simulink model "can_simple_block_bu11143"  (R2016b)
settings: Solver=FixedStepDiscrete  StartTime=0.0  StopTime=1000  FixedStep=0.2  RelTol=1e-3  EnableMultiTasking=on
undefined symbols (not defined in the file or in its folder): A, A10, A14, B, B11, B12, B13, B8, C, CS0, CS1, D, D11, D4, F3, F4, G, G3, G4, H3, H4, K17, K4, L3, N16, PA11, PA12, PD0, PE14, PE15, R10, R14, R17, SCK, SIN, SOUT, T14
libraries: rappid_564xl_ec_toolbox x59
(part 1 of 6)
settings Model: Creator=RMuradov  LastModifiedBy=eugkim01
settings SolverCC: AutoInsertRateTranBlk=on
settings DataIOCC: ExternalInput=off  InitialState=off  LimitDataPoints=on  SaveFormat=Array  SignalLoggingSaveFormat=ModelDataLogs  SaveOutput=off  SignalLogging=off  SaveTime=off
settings OptimizationCC: DefaultParameterBehavior=Inlined  UseDivisionForNetSlopeComputation=on  UseFloatMulNetSlope=on  UseSpecifiedMinMax=on  InlineInvariantSignals=on  PassReuseOutputArgsAs=Individual arguments  ExpressionDepthLimit=2147483647  ZeroExternalMemoryAtStartup=off  ZeroInternalMemoryAtStartup=off  NoFixptDivByZeroProtection=on  EfficientFloat2IntCast=on  LifeSpan=1
settings DebuggingCC: UnderspecifiedInitializationDetection=Classic  MergeDetectMultiDrivingBlocksExec=none  SolverPrmCheckMsg=warning  InheritedTsInSrcMsg=none  SingleTaskRateTransMsg=error  ParameterTunabilityLossMsg=error  FcnCallInpInsideContextMsg=warning  UnconnectedInputMsg=error  UnconnectedOutputMsg=error  UnconnectedLineMsg=error  UnknownTsInhSupMsg=error  StateNameClashWarn=warning  SFUnexpectedBacktrackingDiag=warning  SFNoUnconditionalDefaultTransitionDiag=warning  SFExecutionAtInitializationDiag=none
settings HardwareCC: ProdBitPerPointer=32  ProdBitPerSizeT=32  ProdBitPerPtrDiffT=32  ProdLargestAtomicInteger=Long  ProdLargestAtomicFloat=Double  ProdEndianess=BigEndian  ProdWordSize=32  ProdHWDeviceType=Freescale->32-bit PowerPC
settings ModelReferenceCC: PropagateSignalLabelsOutOfModel=off
settings RTWCC: SystemTargetFile=rappid564xl.tlc  MakeCommand=rappid_564xl_make_rtw  TemplateMakefile=rappid_564xl_default_tmf  PostCodeGenCommand=rappid_analyzegencode(buildInfo)  Description=RAppID Toolbox MPC564xL Code Generation Target (rappid)  GenerateReport=on  TLCAssert=on  BuildConfiguration=Faster Runs  IncludeHyperlinkInReport=on  LaunchReport=on  GenerateTraceInfo=on  GenerateTraceReport=on  GenerateTraceReportSl=on  GenerateTraceReportSf=on  GenerateTraceReportEml=on  GenerateCodeMetricsReport=on
settings CodeAppCC: ForceParamTrailComments=on  IgnoreCustomStorageClasses=off  OperatorAnnotations=on  SimulinkDataObjDesc=on  SFDataObjDesc=on  MATLABFcnDesc=on  CustomSymbolStrGlobalVar=rt$N$M  CustomSymbolStrType=$N$M  CustomSymbolStrFcn=$N$M$F  CustomSymbolStrMacro=$N$M  InsertBlockDesc=on  MATLABSourceComments=on  InternalIdentifier=Classic
settings STFCustomTargetCC: CombineOutputUpdateFcns=on  CombineSignalStateStructs=on  SuppressErrorStatus=on  ERTCustomFileBanners=on  SupportAbsoluteTime=off  SupportNonFinite=off  SupportComplex=off  SupportContinuousTime=off  RemoveResetFunc=on  SupportVariableSizeSignals=on  MATLABClassNameForMDSCustomization=Simulink.SoftwareTarget.ERTCustomization  GRTInterface=off  SystemTargetFile=rappid564xl.tlc
settings ERTTargetCC: ParMdlRefBuildCompliant=off  CompOptLevelCompliant=off  ConcurrentExecutionCompliant=off  CombineSignalStateStructs=on  SuppressErrorStatus=on  ERTFirstTimeCompliant=off  SupportAbsoluteTime=off  SupportNonFinite=off  SupportComplex=off  SupportNonInlinedSFcns=on  SupportVariableSizeSignals=on  ModelStepFunctionPrototypeControlCompliant=off  CPPClassGenCompliant=off  UseToolchainInfoCompliant=off  InlinedParameterPlacement=NonHierarchical  ERTCustomFileTemplate=example_file_process.tlc
settings ConfigComp: CovMetricSettings=dw  CovHtmlReporting=on  CovSaveCumulativeToWorkspaceVar=on  CovSaveSingleToWorkspaceVar=on  CovExternalEMLEnable=off

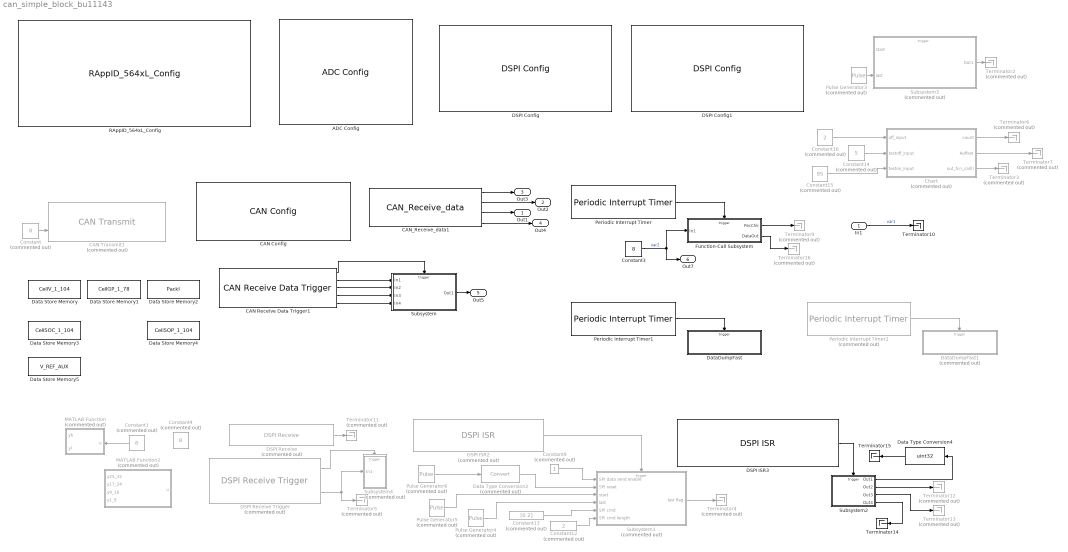
== system can_simple_block_bu11143 ==
  In1 : Inport
  ADC Config : rappid_564xl_ec_toolbox/MPC564xL/Motor Control Blocks/ADC Config  adc_unit=0  adc_ctu=off  adc_owr=on  adc_wls=Left  adc_clk=on  adc_ack=on  adc_ctr0_inp=off  adc_ctr0_shft=10 - Avin = 0  adc_ctr0_cmp=01  adc_ctr0_samp=3  adc_ctr1_inp=off  adc_ctr1_cmp=01  adc_ctr1_samp=1  adc_ctr1_tsens=PTAT  adc_pscr_preval=V0  adc_pscr_preconv=off
  CAN Config : rappid_564xl_ec_toolbox/MPC564xL/Communication Blocks/CAN Config  Priority=1  can_unit=A  can_unit_v2=0  can_idam=A - One full ID (standard or extended) per filter element.  can_srx_dis=1 - Self reception disabled  can_presdiv=4  can_rjw=3  can_pseg1=3  can_pseg2=3  can_clk_src=0 - The CAN engine clock source is the oscillator clock  can_lpb=0 - Loop Back disabled  can_smp=1 - Three samples are used to determine the value of the received bit  can_boff_rec=0 - Automatic recovering from Bus Off state enabled  can_tsyn=0 - Timer Sync feature disabled  can_lbuf=0 - Buffer with highest priority is transmitted first  can_lom=0 - Listen Only Mode is deactivated  can_propseg=6
  CAN Receive Data Trigger1 : rappid_564xl_ec_toolbox/MPC564xL/Communication Blocks/CAN Receive Data Trigger  can_unit=A  can_unit_v2=0  can_buffer=5  can_id=1021  can_isr_prio=14
  CAN Transmit1 : rappid_564xl_ec_toolbox/MPC564xL/Communication Blocks/CAN Transmit  Commented=on  can_unit=A  can_unit_v2=0  can_buffer=14  can_id=522
  CAN_Receive_data1 : rappid_564xl_ec_toolbox/MPC564xL/Communication Blocks/CAN_Receive_data  can_unit=A  can_unit_v2=0  can_buffer=7  can_id=1010
  Chart : Stateflow chart  Commented=on  TreatAsAtomicUnit=on
  Constant : Constant  Commented=on  Value=8  OutDataTypeStr=uint8
  Constant1 : Constant  Commented=on  Value=8  OutDataTypeStr=uint16
  Constant12 : Constant  Commented=on  Value=2  OutDataTypeStr=uint8
  Constant13 : Constant  Commented=on  Value=[0 2]  OutDataTypeStr=uint8
  Constant14 : Constant  Commented=on  Value=5
  Constant15 : Constant  Commented=on  Value=95
  Constant16 : Constant  Commented=on  Value=2
  Constant3 : Constant  Value=8  OutDataTypeStr=uint16
  Constant4 : Constant  Commented=on  Value=8  OutDataTypeStr=uint16
  Constant9 : Constant  Commented=on  OutDataTypeStr=boolean
  DSPI Config : rappid_564xl_ec_toolbox/MPC564xL/Communication Blocks/DSPI Config  Priority=1  dspi_Num=1  dspi_Mode=Master  dspi_MTFE=off  dspi_CONT_SCKE=off  dspi_PCSSE=off  dspi_ROOE=off  dspi_DIS_TXF=Disable  dspi_DIS_RXF_v2=Disable  dspi_SMPL_PT=DSPI samples SIN at driving SCK edge  dspi_FMSZ=8  dspi_CPOL=High  dspi_CPHA=Data is changed on the leading edge of SCK and captured on the following edge  dspi_LSBFE=MSB first  dspi_DBR=off  dspi_PCSSCK=7  dspi_PASC=1  dspi_PDT=5  dspi_PBR=3  dspi_CSSCK=256  dspi_ASC=256  dspi_DT=8  dspi_BR=64  dspi_PCSIS0=High  dspi_PCSIS1=High  dspi_PCSIS2=High  dspi_PCSIS3=High  dspi_PCSIS4=High  dspi_PCSIS5=High  dspi_PCSIS6=High  dspi_PCSIS7=High  dspi_DIS_RXF=Oops
  DSPI Config1 : rappid_564xl_ec_toolbox/MPC564xL/Communication Blocks/DSPI Config  Priority=1  dspi_Num=0  dspi_Mode=Master  dspi_MTFE=off  dspi_CONT_SCKE=off  dspi_PCSSE=off  dspi_ROOE=off  dspi_DIS_TXF=Disable  dspi_DIS_RXF_v2=Disable  dspi_SMPL_PT=DSPI samples SIN at driving SCK edge  dspi_FMSZ=8  dspi_CPOL=High  dspi_CPHA=Data is changed on the leading edge of SCK and captured on the following edge  dspi_LSBFE=MSB first  dspi_DBR=off  dspi_PCSSCK=7  dspi_PASC=1  dspi_PDT=5  dspi_PBR=3  dspi_CSSCK=256  dspi_ASC=256  dspi_DT=8  dspi_BR=64  dspi_PCSIS0=High  dspi_PCSIS1=High  dspi_PCSIS2=High  dspi_PCSIS3=High  dspi_PCSIS4=High  dspi_PCSIS5=High  dspi_PCSIS6=High  dspi_PCSIS7=High  dspi_DIS_RXF=Oops
  DSPI ISR2 : rappid_564xl_ec_toolbox/MPC564xL/Communication Blocks/DSPI ISR  Commented=on  dspi_Num=1  dspi_isr_name=TCF - Transfer Complete  dspi_isrPrio=13  dspi_isr_tfuf=off  dspi_isr_rfof=on
  DSPI ISR3 : rappid_564xl_ec_toolbox/MPC564xL/Communication Blocks/DSPI ISR  dspi_Num=1  dspi_isr_name=EOQF - End of Queue  dspi_isrPrio=11  dspi_isr_tfuf=off  dspi_isr_rfof=on
  DSPI Receive : rappid_564xl_ec_toolbox/MPC564xL/Communication Blocks/DSPI Receive  Commented=on  dspi_Num=1
  DSPI Receive Trigger : rappid_564xl_ec_toolbox/MPC564xL/Communication Blocks/DSPI Receive Trigger  Commented=on  dspi_Num=1  dspi_ISRPri=13
  Data Store Memory : DataStoreMemory  DataStoreName=CellV_1_104  ReadBeforeWriteMsg=warning  WriteAfterWriteMsg=warning  WriteAfterReadMsg=warning  ShowAdditionalParam=off  OutDataTypeStr=uint16  Dimensions=104
  Data Store Memory1 : DataStoreMemory  DataStoreName=CellGP_1_78  ReadBeforeWriteMsg=warning  WriteAfterWriteMsg=warning  WriteAfterReadMsg=warning  ShowAdditionalParam=off  OutDataTypeStr=uint16  Dimensions=78
  Data Store Memory2 : DataStoreMemory  DataStoreName=PackI  ReadBeforeWriteMsg=warning  WriteAfterWriteMsg=warning  WriteAfterReadMsg=warning  ShowAdditionalParam=off  OutDataTypeStr=int32  Dimensions=1
  Data Store Memory3 : DataStoreMemory  DataStoreName=CellSOC_1_104  ReadBeforeWriteMsg=warning  WriteAfterWriteMsg=warning  WriteAfterReadMsg=warning  ShowAdditionalParam=off  OutDataTypeStr=uint16  Dimensions=104
  Data Store Memory4 : DataStoreMemory  DataStoreName=CellSOP_1_104  ReadBeforeWriteMsg=warning  WriteAfterWriteMsg=warning  WriteAfterReadMsg=warning  ShowAdditionalParam=off  OutDataTypeStr=int16  Dimensions=104
  Data Store Memory5 : DataStoreMemory  DataStoreName=V_REF_AUX  ReadBeforeWriteMsg=warning  WriteAfterWriteMsg=warning  WriteAfterReadMsg=warning  InitialValue=3  ShowAdditionalParam=off  OutDataTypeStr=uint16  Dimensions=1
  Data Type Conversion2 : DataTypeConversion  Priority=1  Commented=on
  Data Type Conversion4 : DataTypeConversion  Priority=1  OutDataTypeStr=uint32
  DataDumpFast : Subsystem  TreatAsAtomicUnit=on
      settings: RTWSystemCode=Nonreusable function
  DataDumpFast1 : Subsystem  Commented=on  TreatAsAtomicUnit=on
      settings: RTWSystemCode=Nonreusable function
  Function-Call Subsystem : Subsystem  TreatAsAtomicUnit=on
      settings: RTWSystemCode=Nonreusable function
  MATLAB Function : MATLAB Function  Commented=on  TreatAsAtomicUnit=on
  MATLAB Function2 : MATLAB Function  Commented=on  TreatAsAtomicUnit=on
  Periodic Interrupt Timer : rappid_564xl_ec_toolbox/MPC564xL/General Purpose Blocks/Periodic Interrupt Timer  pit_chan=1  pit_timeout=50  int_priority=12  pit_timeout_val=5999999
  Periodic Interrupt Timer1 : rappid_564xl_ec_toolbox/MPC564xL/General Purpose Blocks/Periodic Interrupt Timer  pit_chan=2  pit_timeout=10  int_priority=13  pit_timeout_val=1199999
  Periodic Interrupt Timer2 : rappid_564xl_ec_toolbox/MPC564xL/General Purpose Blocks/Periodic Interrupt Timer  Commented=on  pit_chan=2  pit_timeout=100  int_priority=13  pit_timeout_val=11999999
  Pulse Generator3 : DiscretePulseGenerator  Commented=on  Period=100  PhaseDelay=5
  Pulse Generator4 : DiscretePulseGenerator  Commented=on  Period=100  PhaseDelay=5
  Pulse Generator5 : DiscretePulseGenerator  Commented=on  Period=100
  Pulse Generator6 : DiscretePulseGenerator  Commented=on  Period=10000000  PhaseDelay=1
  RAppID_564xL_Config : rappid_564xl_ec_toolbox/MPC564xL/RAppID_564xL_Config  SystemClock=120  XTAL=40  MC_clock_60=12  MC_clock_80=16  MC_clock_120=10  SWG_clock_60=20  SWG_clock_80=13.334  SWG_clock_120=20  Compiler=CodeWarrior  MemTarget=FLASH  Part=MPC5643L  Package=144 LQFP  global_int_priority=11  base_tick_priority=12  sys_task_supress=off  exception_handlers=off  stored_mdl_name=can_simple_block_bu11142  freemaster_interface=Oops  freemaster_rx_pin="LINFlex_0 Rx Pin 116 : \"PB[3]\""  freemaster_tx_pin="LINFlex_0 Tx Pin 114 : \"PB[2]\""  freemaster_interface_1=None  freemaster_enable=off  freemaster_rate=57600  freemaster_tx0_pin=18 : B[2] : 114 : A14  freemaster_rx0_pin=19 : B[3] : 116 : B13  freemaster_tx1_pin=57 : D[9] : 26 : L3  freemaster_rx1_pin=29 : B[13] : 60 : R10  freemaster_can_channel=1CH  freemater_can_speed=500K  freemaster_can_msgig=0x7AA  ccp_interface=None  ccp_enable=off  ccp_can_channel=CH1 (MB 0 - 1)  ccp_can_speed=500K  ccp_can_cro_id=256  ccp_can_dto_id=257  ccp_dev_id=RappID  ccp_dev_addr=0  ccp_odt=3  ccp_daq=3  pil_enable=off  pil_bam=off  comport=6  pil_rate=57600  bam_password_def=on  bam_password=0xFEEDFACECAFEBEEF  bam_sa_cs=on  bam_start_address=0x40005000  bam_code_size=0xa000  cons_dspi=on  cons_can=on  cons_adc=on  cons_pwm=on  cons_ctu=on  cons_swg=on  cons_eTimer=on  cons_fm=on
  Subsystem : Subsystem
      settings: RTWSystemCode=Nonreusable function
  Subsystem1 : Subsystem  Commented=on
      settings: RTWSystemCode=Nonreusable function
  Subsystem2 : Subsystem
      settings: RTWSystemCode=Nonreusable function
  Subsystem3 : Subsystem  Commented=on
  Subsystem4 : Subsystem  Commented=on
      settings: RTWSystemCode=Nonreusable function
  Terminator10 : Terminator
  Terminator{2..7,9,11..13,16} (11 alike) : Terminator  Commented=on
  Terminator14 : Terminator
  Terminator15 : Terminator
  Out1 : Outport
  Out2 : Outport  Port=2
  Out3 : Outport  Port=3
  Out4 : Outport  Port=4
  Out5 : Outport  Port=5
  Out7 : Outport  Port=6
  wires:
  CAN_Receive_data1/4 -> Out4/1
  CAN_Receive_data1/3 -> Out1/1
  CAN_Receive_data1/2 -> Out2/1
  CAN_Receive_data1/1 -> Out3/1
  Constant/1 -> CAN Transmit1/2
  CAN Receive Data Trigger1/3 -> Subsystem/2(In2)
  CAN Receive Data Trigger1/4 -> Subsystem/3(In3)
  CAN Receive Data Trigger1/5 -> Subsystem/4(In4)
  CAN Receive Data Trigger1/2 -> Subsystem/1(In1)
  CAN Receive Data Trigger1/1 -> Subsystem/Trigger
  Subsystem/1(Out1) -> Out5/1
  DSPI ISR2/1 -> Subsystem1/Trigger
  DSPI ISR3/1 -> Subsystem2/Trigger
  Constant9/1 -> Subsystem1/1(SPI data send enable)
  Subsystem1/1(last flag) -> Terminator4/1
  Pulse Generator3/1 -> Subsystem3/2(last)
  Subsystem3/1(Out1) -> Terminator2/1
  Pulse Generator4/1 -> Subsystem1/4(last)
  Constant12/1 -> Subsystem1/6(SPI cmd length)
  Constant13/1 -> Subsystem1/5(SPI cmd)
  Chart/1(count) -> Terminator6/1
  Chart/2(" Aoffset") -> Terminator7/1
  Constant16/1 -> Chart/1(off_input)
  Constant14/1 -> Chart/2(testoff_input)
  Constant15/1 -> Chart/3(teston_input)
  Pulse Generator5/1 -> Subsystem1/3(start)
  Pulse Generator6/1 -> Data Type Conversion2/1
  Data Type Conversion2/1 -> Subsystem1/2(SPI reset)
  Chart/3(out_fcn_call()) -> Terminator3/1
  Periodic Interrupt Timer/1 -> Function-Call Subsystem/Trigger
  In1/1 -> Terminator10/1  "var1"
  Constant3/1 -> Function-Call Subsystem/1(In1), Out7/1  "var2"
  Data Type Conversion4/1 -> Terminator15/1
  DSPI Receive Trigger/2 -> Terminator5/1, Subsystem4/1(In1)
  DSPI Receive Trigger/1 -> Subsystem4/Trigger
  Subsystem2/1(Out1) -> Data Type Conversion4/1
  DSPI Receive/1 -> Terminator11/1
  Subsystem2/4(Out4) -> Terminator14/1
  Subsystem2/2(Out2) -> Terminator12/1
  Subsystem2/3(Out3) -> Terminator13/1
  Constant1/1 -> MATLAB Function/1(u)
  Function-Call Subsystem/1(PecChk) -> Terminator9/1
  Function-Call Subsystem/2(DataOut) -> Terminator16/1
  Periodic Interrupt Timer1/1 -> DataDumpFast/Trigger
  Periodic Interrupt Timer2/1 -> DataDumpFast1/Trigger

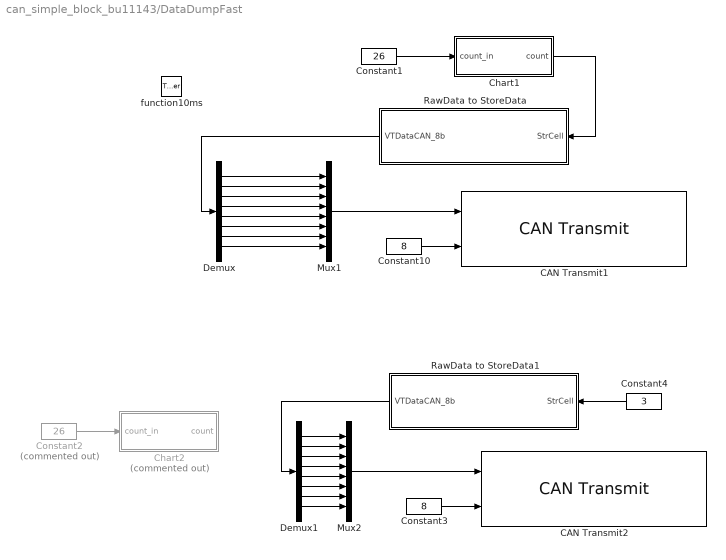
== system can_simple_block_bu11143/DataDumpFast ==
  function10ms : TriggerPort  TriggerType=function-call  VariantControl=Variant
  CAN Transmit1 : rappid_564xl_ec_toolbox/MPC564xL/Communication Blocks/CAN Transmit  can_unit=A  can_unit_v2=0  can_buffer=26  can_id=522
  CAN Transmit2 : rappid_564xl_ec_toolbox/MPC564xL/Communication Blocks/CAN Transmit  can_unit=A  can_unit_v2=0  can_buffer=27  can_id=523
  Chart1 : Stateflow chart  TreatAsAtomicUnit=on
  Chart2 : Stateflow chart  Commented=on  TreatAsAtomicUnit=on
  Constant1 : Constant  Value=26  OutDataTypeStr=uint8
  Constant10 : Constant  Value=8  OutDataTypeStr=uint8
  Constant2 : Constant  Commented=on  Value=26  OutDataTypeStr=uint8
  Constant3 : Constant  Value=8  OutDataTypeStr=uint8
  Constant4 : Constant  Value=3  OutDataTypeStr=uint8
  Demux : Demux  Outputs=8
  Demux1 : Demux  Outputs=8
  Mux1 : Mux  Inputs=8
  Mux2 : Mux  Inputs=8
  RawData to StoreData : MATLAB Function  TreatAsAtomicUnit=on
  RawData to StoreData1 : MATLAB Function  TreatAsAtomicUnit=on
  wires:
  Constant10/1 -> CAN Transmit1/2
  RawData to StoreData/1(VTDataCAN_8b) -> Demux/1
  Constant1/1 -> Chart1/1(count_in)
  Chart1/1(count) -> RawData to StoreData/1(StrCell)
  Demux/1 -> Mux1/1
  Demux/2 -> Mux1/2
  Demux/3 -> Mux1/3
  Demux/4 -> Mux1/4
  Demux/5 -> Mux1/5
  Demux/6 -> Mux1/6
  Demux/8 -> Mux1/8
  Demux/7 -> Mux1/7
  Mux1/1 -> CAN Transmit1/1
  Constant3/1 -> CAN Transmit2/2
  RawData to StoreData1/1(VTDataCAN_8b) -> Demux1/1
  Constant4/1 -> RawData to StoreData1/1(StrCell)
  Demux1/1 -> Mux2/1
  Demux1/2 -> Mux2/2
  Demux1/3 -> Mux2/3
  Demux1/4 -> Mux2/4
  Demux1/5 -> Mux2/5
  Demux1/6 -> Mux2/6
  Demux1/8 -> Mux2/8
  Demux1/7 -> Mux2/7
  Mux2/1 -> CAN Transmit2/1
  Constant2/1 -> Chart2/1(count_in)

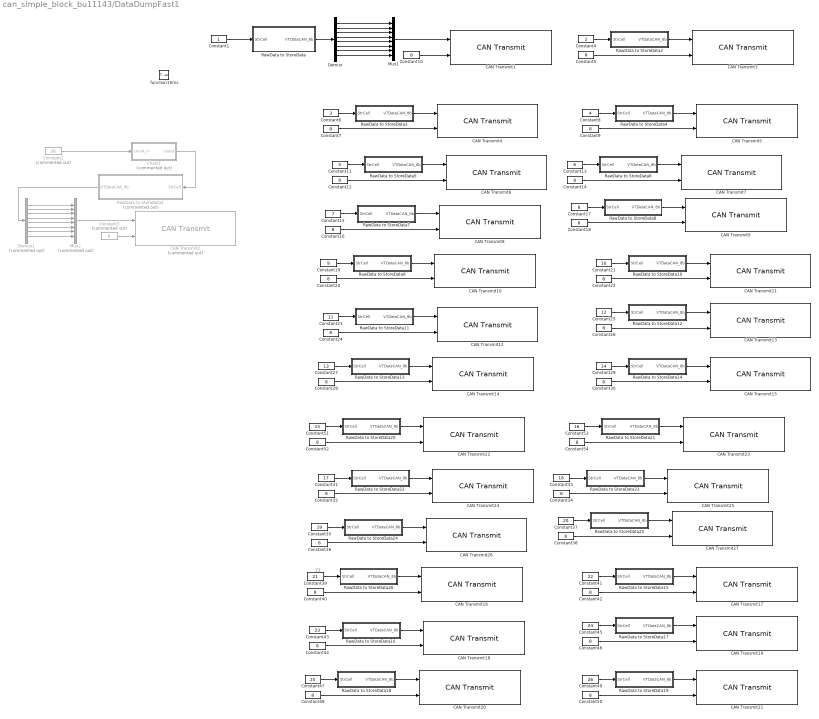
== system can_simple_block_bu11143/DataDumpFast1 ==
  note: 21
  function10ms : TriggerPort  TriggerType=function-call  VariantControl=Variant
  CAN Transmit1 : rappid_564xl_ec_toolbox/MPC564xL/Communication Blocks/CAN Transmit  can_unit=A  can_unit_v2=0  can_buffer=0  can_id=530
  CAN Transmit10 : rappid_564xl_ec_toolbox/MPC564xL/Communication Blocks/CAN Transmit  can_unit=A  can_unit_v2=0  can_buffer=8  can_id=538
  CAN Transmit11 : rappid_564xl_ec_toolbox/MPC564xL/Communication Blocks/CAN Transmit  can_unit=A  can_unit_v2=0  can_buffer=9  can_id=539
  CAN Transmit12 : rappid_564xl_ec_toolbox/MPC564xL/Communication Blocks/CAN Transmit  can_unit=A  can_unit_v2=0  can_buffer=10  can_id=540
  CAN Transmit13 : rappid_564xl_ec_toolbox/MPC564xL/Communication Blocks/CAN Transmit  can_unit=A  can_unit_v2=0  can_buffer=11  can_id=541
  CAN Transmit14 : rappid_564xl_ec_toolbox/MPC564xL/Communication Blocks/CAN Transmit  can_unit=A  can_unit_v2=0  can_buffer=12  can_id=542
  CAN Transmit15 : rappid_564xl_ec_toolbox/MPC564xL/Communication Blocks/CAN Transmit  can_unit=A  can_unit_v2=0  can_buffer=13  can_id=543
  CAN Transmit16 : rappid_564xl_ec_toolbox/MPC564xL/Communication Blocks/CAN Transmit  can_unit=A  can_unit_v2=0  can_buffer=20  can_id=550
  CAN Transmit17 : rappid_564xl_ec_toolbox/MPC564xL/Communication Blocks/CAN Transmit  can_unit=A  can_unit_v2=0  can_buffer=21  can_id=551
  CAN Transmit18 : rappid_564xl_ec_toolbox/MPC564xL/Communication Blocks/CAN Transmit  can_unit=A  can_unit_v2=0  can_buffer=22  can_id=552
  CAN Transmit19 : rappid_564xl_ec_toolbox/MPC564xL/Communication Blocks/CAN Transmit  can_unit=A  can_unit_v2=0  can_buffer=23  can_id=553
  CAN Transmit2 : rappid_564xl_ec_toolbox/MPC564xL/Communication Blocks/CAN Transmit  Commented=on  can_unit=A  can_unit_v2=0  can_buffer=15  can_id=523
  CAN Transmit20 : rappid_564xl_ec_toolbox/MPC564xL/Communication Blocks/CAN Transmit  can_unit=A  can_unit_v2=0  can_buffer=24  can_id=554
  CAN Transmit21 : rappid_564xl_ec_toolbox/MPC564xL/Communication Blocks/CAN Transmit  can_unit=A  can_unit_v2=0  can_buffer=25  can_id=555
  CAN Transmit22 : rappid_564xl_ec_toolbox/MPC564xL/Communication Blocks/CAN Transmit  can_unit=A  can_unit_v2=0  can_buffer=14  can_id=544
  CAN Transmit23 : rappid_564xl_ec_toolbox/MPC564xL/Communication Blocks/CAN Transmit  can_unit=A  can_unit_v2=0  can_buffer=15  can_id=545
  CAN Transmit24 : rappid_564xl_ec_toolbox/MPC564xL/Communication Blocks/CAN Transmit  can_unit=A  can_unit_v2=0  can_buffer=16  can_id=546
  CAN Transmit25 : rappid_564xl_ec_toolbox/MPC564xL/Communication Blocks/CAN Transmit  can_unit=A  can_unit_v2=0  can_buffer=17  can_id=547
  CAN Transmit26 : rappid_564xl_ec_toolbox/MPC564xL/Communication Blocks/CAN Transmit  can_unit=A  can_unit_v2=0  can_buffer=18  can_id=548
  CAN Transmit27 : rappid_564xl_ec_toolbox/MPC564xL/Communication Blocks/CAN Transmit  can_unit=A  can_unit_v2=0  can_buffer=19  can_id=549
  CAN Transmit3 : rappid_564xl_ec_toolbox/MPC564xL/Communication Blocks/CAN Transmit  can_unit=A  can_unit_v2=0  can_buffer=1  can_id=531
  CAN Transmit4 : rappid_564xl_ec_toolbox/MPC564xL/Communication Blocks/CAN Transmit  can_unit=A  can_unit_v2=0  can_buffer=2  can_id=532
  CAN Transmit5 : rappid_564xl_ec_toolbox/MPC564xL/Communication Blocks/CAN Transmit  can_unit=A  can_unit_v2=0  can_buffer=3  can_id=533
  CAN Transmit6 : rappid_564xl_ec_toolbox/MPC564xL/Communication Blocks/CAN Transmit  can_unit=A  can_unit_v2=0  can_buffer=4  can_id=534
  CAN Transmit7 : rappid_564xl_ec_toolbox/MPC564xL/Communication Blocks/CAN Transmit  can_unit=A  can_unit_v2=0  can_buffer=5  can_id=535
  CAN Transmit8 : rappid_564xl_ec_toolbox/MPC564xL/Communication Blocks/CAN Transmit  can_unit=A  can_unit_v2=0  can_buffer=6  can_id=536
  CAN Transmit9 : rappid_564xl_ec_toolbox/MPC564xL/Communication Blocks/CAN Transmit  can_unit=A  can_unit_v2=0  can_buffer=7  can_id=537
  Chart2 : Stateflow chart  Commented=on  TreatAsAtomicUnit=on
  Constant1 : Constant  OutDataTypeStr=uint8
  Constant{5,7,9..10,12,14,16..18,20,22,24,26,28,30,32,34,36,38,40,42,44,46,48,50,52,54} (27 alike) : Constant  Value=8  OutDataTypeStr=uint8
  Constant11 : Constant  Value=5  OutDataTypeStr=uint8
  Constant13 : Constant  Value=6  OutDataTypeStr=uint8
  Constant15 : Constant  Value=7  OutDataTypeStr=uint8
  Constant19 : Constant  Value=9  OutDataTypeStr=uint8
  Constant2 : Constant  Commented=on  Value=26  OutDataTypeStr=uint8
  Constant21 : Constant  Value=10  OutDataTypeStr=uint8
  Constant23 : Constant  Value=11  OutDataTypeStr=uint8
  Constant25 : Constant  Value=12  OutDataTypeStr=uint8
  Constant27 : Constant  Value=13  OutDataTypeStr=uint8
  Constant29 : Constant  Value=14  OutDataTypeStr=uint8
  Constant3 : Constant  Commented=on  Value=8  OutDataTypeStr=uint8
  Constant31 : Constant  Value=17  OutDataTypeStr=uint8
  Constant33 : Constant  Value=18  OutDataTypeStr=uint8
  Constant35 : Constant  Value=19  OutDataTypeStr=uint8
  Constant37 : Constant  Value=20  OutDataTypeStr=uint8
  Constant39 : Constant  Value=21  OutDataTypeStr=uint8
  Constant4 : Constant  Value=2  OutDataTypeStr=uint8
  Constant41 : Constant  Value=22  OutDataTypeStr=uint8
  Constant43 : Constant  Value=23  OutDataTypeStr=uint8
  Constant45 : Constant  Value=24  OutDataTypeStr=uint8
  Constant47 : Constant  Value=25  OutDataTypeStr=uint8
  Constant49 : Constant  Value=26  OutDataTypeStr=uint8
  Constant51 : Constant  Value=15  OutDataTypeStr=uint8
  Constant53 : Constant  Value=16  OutDataTypeStr=uint8
  Constant6 : Constant  Value=3  OutDataTypeStr=uint8
  Constant8 : Constant  Value=4  OutDataTypeStr=uint8
  Demux : Demux  Outputs=8
  Demux1 : Demux  Commented=on  Outputs=8
  Mux1 : Mux  Inputs=8
  Mux2 : Mux  Commented=on  Inputs=8
  RawData to StoreData : MATLAB Function  TreatAsAtomicUnit=on
  RawData to StoreData1 : MATLAB Function  Commented=on  TreatAsAtomicUnit=on
  RawData to StoreData10 : MATLAB Function  TreatAsAtomicUnit=on
  RawData to StoreData11 : MATLAB Function  TreatAsAtomicUnit=on
  RawData to StoreData12 : MATLAB Function  TreatAsAtomicUnit=on
  RawData to StoreData13 : MATLAB Function  TreatAsAtomicUnit=on
  RawData to StoreData14 : MATLAB Function  TreatAsAtomicUnit=on
  RawData to StoreData15 : MATLAB Function  TreatAsAtomicUnit=on
  RawData to StoreData16 : MATLAB Function  TreatAsAtomicUnit=on
  RawData to StoreData17 : MATLAB Function  TreatAsAtomicUnit=on
  RawData to StoreData18 : MATLAB Function  TreatAsAtomicUnit=on
  RawData to StoreData19 : MATLAB Function  TreatAsAtomicUnit=on
  RawData to StoreData2 : MATLAB Function  TreatAsAtomicUnit=on
  RawData to StoreData20 : MATLAB Function  TreatAsAtomicUnit=on
  RawData to StoreData21 : MATLAB Function  TreatAsAtomicUnit=on
  RawData to StoreData22 : MATLAB Function  TreatAsAtomicUnit=on
  RawData to StoreData23 : MATLAB Function  TreatAsAtomicUnit=on
  RawData to StoreData24 : MATLAB Function  TreatAsAtomicUnit=on
  RawData to StoreData25 : MATLAB Function  TreatAsAtomicUnit=on
  RawData to StoreData26 : MATLAB Function  TreatAsAtomicUnit=on
  RawData to StoreData3 : MATLAB Function  TreatAsAtomicUnit=on
  RawData to StoreData4 : MATLAB Function  TreatAsAtomicUnit=on
  RawData to StoreData5 : MATLAB Function  TreatAsAtomicUnit=on
  RawData to StoreData6 : MATLAB Function  TreatAsAtomicUnit=on
  RawData to StoreData7 : MATLAB Function  TreatAsAtomicUnit=on
  RawData to StoreData8 : MATLAB Function  TreatAsAtomicUnit=on
  RawData to StoreData9 : MATLAB Function  TreatAsAtomicUnit=on
  wires:
  Constant10/1 -> CAN Transmit1/2
  RawData to StoreData/1(VTDataCAN_8b) -> Demux/1
  Constant1/1 -> RawData to StoreData/1(StrCell)
  Demux/1 -> Mux1/1
  Demux/2 -> Mux1/2
  Demux/3 -> Mux1/3
  Demux/4 -> Mux1/4
  Demux/5 -> Mux1/5
  Demux/6 -> Mux1/6
  Demux/8 -> Mux1/8
  Demux/7 -> Mux1/7
  Mux1/1 -> CAN Transmit1/1
  Constant3/1 -> CAN Transmit2/2
  RawData to StoreData1/1(VTDataCAN_8b) -> Demux1/1
  Constant2/1 -> Chart2/1(count_in)
  Chart2/1(count) -> RawData to StoreData1/1(StrCell)
  Demux1/1 -> Mux2/1
  Demux1/2 -> Mux2/2
  Demux1/3 -> Mux2/3
  Demux1/4 -> Mux2/4
  Demux1/5 -> Mux2/5
  Demux1/6 -> Mux2/6
  Demux1/8 -> Mux2/8
  Demux1/7 -> Mux2/7
  Mux2/1 -> CAN Transmit2/1
  Constant4/1 -> RawData to StoreData2/1(StrCell)
  RawData to StoreData2/1(VTDataCAN_8b) -> CAN Transmit3/1
  Constant5/1 -> CAN Transmit3/2
  Constant6/1 -> RawData to StoreData3/1(StrCell)
  RawData to StoreData3/1(VTDataCAN_8b) -> CAN Transmit4/1
  Constant7/1 -> CAN Transmit4/2
  Constant8/1 -> RawData to StoreData4/1(StrCell)
  RawData to StoreData4/1(VTDataCAN_8b) -> CAN Transmit5/1
  Constant9/1 -> CAN Transmit5/2
  Constant11/1 -> RawData to StoreData5/1(StrCell)
  RawData to StoreData5/1(VTDataCAN_8b) -> CAN Transmit6/1
  Constant12/1 -> CAN Transmit6/2
  Constant13/1 -> RawData to StoreData6/1(StrCell)
  RawData to StoreData6/1(VTDataCAN_8b) -> CAN Transmit7/1
  Constant14/1 -> CAN Transmit7/2
  Constant15/1 -> RawData to StoreData7/1(StrCell)
  RawData to StoreData7/1(VTDataCAN_8b) -> CAN Transmit8/1
  Constant16/1 -> CAN Transmit8/2
  Constant17/1 -> RawData to StoreData8/1(StrCell)
  RawData to StoreData8/1(VTDataCAN_8b) -> CAN Transmit9/1
  Constant18/1 -> CAN Transmit9/2
  Constant19/1 -> RawData to StoreData9/1(StrCell)
  RawData to StoreData9/1(VTDataCAN_8b) -> CAN Transmit10/1
  Constant20/1 -> CAN Transmit10/2
  Constant21/1 -> RawData to StoreData10/1(StrCell)
  RawData to StoreData10/1(VTDataCAN_8b) -> CAN Transmit11/1
  Constant22/1 -> CAN Transmit11/2
  Constant23/1 -> RawData to StoreData11/1(StrCell)
  RawData to StoreData11/1(VTDataCAN_8b) -> CAN Transmit12/1
  Constant24/1 -> CAN Transmit12/2
  Constant25/1 -> RawData to StoreData12/1(StrCell)
  RawData to StoreData12/1(VTDataCAN_8b) -> CAN Transmit13/1
  Constant26/1 -> CAN Transmit13/2
  Constant27/1 -> RawData to StoreData13/1(StrCell)
  RawData to StoreData13/1(VTDataCAN_8b) -> CAN Transmit14/1
  Constant28/1 -> CAN Transmit14/2
  Constant29/1 -> RawData to StoreData14/1(StrCell)
  RawData to StoreData14/1(VTDataCAN_8b) -> CAN Transmit15/1
  Constant30/1 -> CAN Transmit15/2
  Constant51/1 -> RawData to StoreData20/1(StrCell)
  RawData to StoreData20/1(VTDataCAN_8b) -> CAN Transmit22/1
  Constant52/1 -> CAN Transmit22/2
  Constant53/1 -> RawData to StoreData21/1(StrCell)
  RawData to StoreData21/1(VTDataCAN_8b) -> CAN Transmit23/1
  Constant54/1 -> CAN Transmit23/2
  Constant31/1 -> RawData to StoreData22/1(StrCell)
  RawData to StoreData22/1(VTDataCAN_8b) -> CAN Transmit24/1
  Constant32/1 -> CAN Transmit24/2
  Constant33/1 -> RawData to StoreData23/1(StrCell)
  RawData to StoreData23/1(VTDataCAN_8b) -> CAN Transmit25/1
  Constant34/1 -> CAN Transmit25/2
  Constant35/1 -> RawData to StoreData24/1(StrCell)
  RawData to StoreData24/1(VTDataCAN_8b) -> CAN Transmit26/1
  Constant36/1 -> CAN Transmit26/2
  Constant37/1 -> RawData to StoreData25/1(StrCell)
  RawData to StoreData25/1(VTDataCAN_8b) -> CAN Transmit27/1
  Constant38/1 -> CAN Transmit27/2
  Constant39/1 -> RawData to StoreData26/1(StrCell)
  RawData to StoreData26/1(VTDataCAN_8b) -> CAN Transmit16/1
  Constant40/1 -> CAN Transmit16/2
  Constant41/1 -> RawData to StoreData15/1(StrCell)
  RawData to StoreData15/1(VTDataCAN_8b) -> CAN Transmit17/1
  Constant42/1 -> CAN Transmit17/2
  Constant43/1 -> RawData to StoreData16/1(StrCell)
  RawData to StoreData16/1(VTDataCAN_8b) -> CAN Transmit18/1
  Constant44/1 -> CAN Transmit18/2
  Constant45/1 -> RawData to StoreData17/1(StrCell)
  RawData to StoreData17/1(VTDataCAN_8b) -> CAN Transmit19/1
  Constant46/1 -> CAN Transmit19/2
  Constant47/1 -> RawData to StoreData18/1(StrCell)
  RawData to StoreData18/1(VTDataCAN_8b) -> CAN Transmit20/1
  Constant48/1 -> CAN Transmit20/2
  Constant49/1 -> RawData to StoreData19/1(StrCell)
  RawData to StoreData19/1(VTDataCAN_8b) -> CAN Transmit21/1
  Constant50/1 -> CAN Transmit21/2

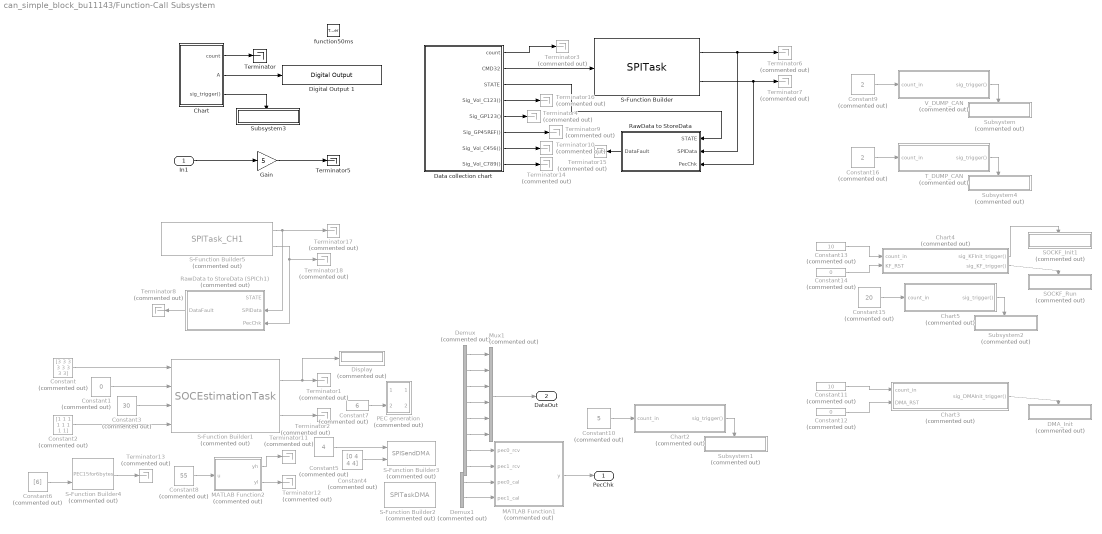
== system can_simple_block_bu11143/Function-Call Subsystem ==
  In1 : Inport
  function50ms : TriggerPort  TriggerType=function-call  VariantControl=Variant
  Chart : Stateflow chart  TreatAsAtomicUnit=on
  Chart2 : Stateflow chart  Commented=on  TreatAsAtomicUnit=on
  Chart3 : Stateflow chart  Commented=on  TreatAsAtomicUnit=on
  Chart4 : Stateflow chart  Commented=on  TreatAsAtomicUnit=on
  Chart5 : Stateflow chart  Commented=on  TreatAsAtomicUnit=on
  Constant : Constant  Commented=on  Value=[3 3 3 3 3 3 3 3]
  Constant1 : Constant  Commented=on  Value=0
  Constant10 : Constant  Commented=on  Value=5  OutDataTypeStr=Inherit: Inherit via back propagation
  Constant11 : Constant  Commented=on  Value=10  OutDataTypeStr=Inherit: Inherit via back propagation
  Constant12 : Constant  Commented=on  Value=0  OutDataTypeStr=Inherit: Inherit via back propagation
  Constant13 : Constant  Commented=on  Value=10  OutDataTypeStr=Inherit: Inherit via back propagation
  Constant14 : Constant  Commented=on  Value=0  OutDataTypeStr=Inherit: Inherit via back propagation
  Constant15 : Constant  Commented=on  Value=20  OutDataTypeStr=Inherit: Inherit via back propagation
  Constant16 : Constant  Commented=on  Value=2  OutDataTypeStr=Inherit: Inherit via back propagation
  Constant2 : Constant  Commented=on  Value=[1 1 1 1 1 1 1 1]  OutDataTypeStr=boolean
  Constant3 : Constant  Commented=on  Value=30
  Constant4 : Constant  Commented=on  Value=[0 4 4 4]  OutDataTypeStr=Inherit: Inherit via back propagation
  Constant5 : Constant  Commented=on  Value=4  OutDataTypeStr=Inherit: Inherit via back propagation
  Constant6 : Constant  Commented=on  Value=[6]  OutDataTypeStr=Inherit: Inherit via back propagation
  Constant7 : Constant  Commented=on  Value=6  OutDataTypeStr=Inherit: Inherit via back propagation
  Constant8 : Constant  Commented=on  Value=55  OutDataTypeStr=Inherit: Inherit via back propagation
  Constant9 : Constant  Commented=on  Value=2  OutDataTypeStr=Inherit: Inherit via back propagation
  DMA_Init : Subsystem  Commented=on
  Data collection chart : Stateflow chart  TreatAsAtomicUnit=on
  Demux : Demux  Commented=on  Outputs=8
  Demux1 : Demux  Commented=on  Outputs=2
  Digital Output 1 : rappid_564xl_ec_toolbox/MPC564xL/General Purpose Blocks/Digital Output   gpio_outputs="78  : PE14 : [ 119 ] : [ B12 ]"  pinNum=[ 119 ]  pcrNum=78
  Display : Display  Commented=on
  Gain : Gain  Gain=5
  MATLAB Function1 : MATLAB Function  Commented=on  TreatAsAtomicUnit=on
  MATLAB Function2 : MATLAB Function  Commented=on  TreatAsAtomicUnit=on
  Mux1 : Mux  Commented=on  Inputs=6
  PEC generation : MATLAB Function  Commented=on  TreatAsAtomicUnit=on
  RawData to StoreData : MATLAB Function  TreatAsAtomicUnit=on
  RawData to StoreData (SPICh1) : MATLAB Function  Commented=on  TreatAsAtomicUnit=on
  S-Function Builder : S-Function  InitFcn=try, set_param(gcb,'FunctionName','SPITask'), end  FunctionName=SPITask  SFunctionModules=SPITask_wrapper BMU_Driver  SFunctionDeploymentMode=off  EnableBusSupport=off  mask(S-Function Builder){}
      mask help: Simulink:masks:SFunctionBuilder_MD
      mask init:
      | val = [[.9  0.75 0.75 1 1 .9 .9 1]',[1 1 0.75 0.75 .9 .9 1 .9]'];try , sys = get_param(gcb,'SfunBuilderFcnName');if isempty(sys), sys = get_param(gcb,'FunctionName'); end,catch, sys = get_param(gcb,'FunctionName'); end
      settings: CopyFcn=set_param(gcbh,'LinkStatus','none')  PreSaveFcn=try, set_param(gcb,'FunctionName','SPITask'), end  OpenFcn=sfunctionwizard(gcbh)
      mask Display:
      | plot(val(:,1),val(:,2))
      | disp(sys)
      | port_label('input',1,'CMD32')
      | port_label('output',1,'y0')
      | port_label('output',2,'PecChk')
  S-Function Builder1 : S-Function  Commented=on  InitFcn=try, set_param(gcb,'FunctionName','SOCEstimationTask'), end  FunctionName=SOCEstimationTask  SFunctionModules=SOCEstimationTask_wrapper Extended look2_binlx rtGetNaN rtGetInf rt_nonfinite const_params  SFunctionDeploymentMode=off  EnableBusSupport=off  mask(S-Function Builder){}
      mask help: Simulink:masks:SFunctionBuilder_MD
      mask init: same as can_simple_block_bu11143/Function-Call Subsystem/S-Function Builder
      settings: CopyFcn=set_param(gcbh,'LinkStatus','none')  PreSaveFcn=try, set_param(gcb,'FunctionName','SOCEstimationTask'), end  OpenFcn=sfunctionwizard(gcbh)
      mask Display: plot(val(:,1),val(:,2)),disp(sys), port_label('input',1,'I'), port_label('input',2,'V8'), port_label('input',3,'T'), port_label('input',4,'Enable8'), port_label('output',1,'SOC'), port_label('output',2,'Vt')
  S-Function Builder2 : S-Function  Commented=on  InitFcn=try, set_param(gcb,'FunctionName','SPITaskDMA'), end  FunctionName=SPITaskDMA  SFunctionModules=SPITaskDMA_wrapper BMU_Driver  SFunctionDeploymentMode=off  EnableBusSupport=off  mask(S-Function Builder){}
      mask help: Simulink:masks:SFunctionBuilder_MD
      mask init: same as can_simple_block_bu11143/Function-Call Subsystem/S-Function Builder
      settings: CopyFcn=set_param(gcbh,'LinkStatus','none')  PreSaveFcn=try, set_param(gcb,'FunctionName','SPITaskDMA'), end  OpenFcn=sfunctionwizard(gcbh)
      mask Display: plot(val(:,1),val(:,2)),disp(sys), port_label('output',1,'y0')
  S-Function Builder3 : S-Function  Commented=on  InitFcn=try, set_param(gcb,'FunctionName','SPISendDMA'), end  FunctionName=SPISendDMA  SFunctionModules=SPISendDMA_wrapper DMA  SFunctionDeploymentMode=off  EnableBusSupport=off  mask(S-Function Builder){}
      mask help: Simulink:masks:SFunctionBuilder_MD
      mask init: same as can_simple_block_bu11143/Function-Call Subsystem/S-Function Builder
      settings: CopyFcn=set_param(gcbh,'LinkStatus','none')  PreSaveFcn=try, set_param(gcb,'FunctionName','SPISendDMA'), end  OpenFcn=sfunctionwizard(gcbh)
      mask Display: plot(val(:,1),val(:,2)),disp(sys), port_label('input',1,'len'), port_label('input',2,'data')
  S-Function Builder4 : S-Function  Commented=on  InitFcn=try, set_param(gcb,'FunctionName','PEC15for6bytes'), end  FunctionName=PEC15for6bytes  SFunctionModules=PEC15for6bytes_wrapper BMU_Driver  SFunctionDeploymentMode=off  EnableBusSupport=off  mask(S-Function Builder){}
      mask help: Simulink:masks:SFunctionBuilder_MD
      mask init: same as can_simple_block_bu11143/Function-Call Subsystem/S-Function Builder
      settings: CopyFcn=set_param(gcbh,'LinkStatus','none')  PreSaveFcn=try, set_param(gcb,'FunctionName','PEC15for6bytes'), end  OpenFcn=sfunctionwizard(gcbh)
      mask Display: plot(val(:,1),val(:,2)),disp(sys), port_label('input',1,'data'), port_label('input',2,'len'), port_label('output',1,'y0')
  S-Function Builder5 : S-Function  Commented=on  InitFcn=try, set_param(gcb,'FunctionName','SPITask_CH1'), end  FunctionName=SPITask_CH1  SFunctionModules=SPITask_CH1_wrapper BMU_Driver  SFunctionDeploymentMode=off  EnableBusSupport=off  mask(S-Function Builder){}
      mask help: Simulink:masks:SFunctionBuilder_MD
      mask init: same as can_simple_block_bu11143/Function-Call Subsystem/S-Function Builder
      settings: CopyFcn=set_param(gcbh,'LinkStatus','none')  PreSaveFcn=try, set_param(gcb,'FunctionName','SPITask_CH1'), end  OpenFcn=sfunctionwizard(gcbh)
      mask Display: plot(val(:,1),val(:,2)),disp(sys), port_label('input',1,'CMD32'), port_label('output',1,'y0'), port_label('output',2,'PecChk')
  SOCKF_Init1 : Subsystem  Commented=on
  SOCKF_Run : Subsystem  Commented=on
  Subsystem : Subsystem  Commented=on
  Subsystem1 : Subsystem  Commented=on
  Subsystem2 : Subsystem  Commented=on
  Subsystem3 : Subsystem
  Subsystem4 : Subsystem  Commented=on
  T_DUMP_CAN : Stateflow chart  Commented=on  TreatAsAtomicUnit=on
  Terminator : Terminator
  Terminator{1..4,6..18} (17 alike) : Terminator  Commented=on
  Terminator5 : Terminator
  V_DUMP_CAN : Stateflow chart  Commented=on  TreatAsAtomicUnit=on
  PecChk : Outport
  DataOut : Outport  Port=2
  wires:
  In1/1 -> Gain/1
  Gain/1 -> Terminator5/1
  Chart/2(" A") -> Digital Output 1/1
  Chart/1(count) -> Terminator/1
  S-Function Builder/1 -> Terminator6/1, RawData to StoreData/2(SPIData)
  S-Function Builder1/1 -> Terminator1/1, Display/1
  S-Function Builder1/2 -> Terminator2/1
  Constant/1 -> S-Function Builder1/1
  Constant1/1 -> S-Function Builder1/2
  Constant2/1 -> S-Function Builder1/4
  Constant3/1 -> S-Function Builder1/3
  Constant4/1 -> S-Function Builder3/2
  Constant5/1 -> S-Function Builder3/1
  Constant6/1 -> S-Function Builder4/2
  Demux/7 -> MATLAB Function1/1(pec0_rcv)
  Demux/8 -> MATLAB Function1/2(pec1_rcv)
  MATLAB Function1/1(y) -> PecChk/1
  Demux/1 -> Mux1/1
  Demux/2 -> Mux1/2
  Demux/3 -> Mux1/3
  Demux/4 -> Mux1/4
  Demux/5 -> Mux1/5
  Demux/6 -> Mux1/6
  S-Function Builder4/1 -> Terminator13/1
  Mux1/1 -> DataOut/1
  Constant7/1 -> PEC generation/2(len)
  MATLAB Function2/1(yh) -> Terminator11/1
  MATLAB Function2/2(yl) -> Terminator12/1
  Constant8/1 -> MATLAB Function2/1(u)
  S-Function Builder/2 -> Terminator7/1, RawData to StoreData/3(PecChk)
  Demux1/1 -> MATLAB Function1/3(pec0_cal)
  Demux1/2 -> MATLAB Function1/4(pec1_cal)
  Data collection chart/1(count) -> Terminator3/1
  Data collection chart/2(CMD32) -> S-Function Builder/1
  Data collection chart/3(STATE) -> RawData to StoreData/1(STATE)
  Data collection chart/5(Sig_GP123()) -> Terminator4/1
  Data collection chart/6(Sig_GP45REF()) -> Terminator9/1
  Data collection chart/7(Sig_Vol_C456()) -> Terminator10/1
  Data collection chart/8(Sig_Vol_C789()) -> Terminator14/1
  RawData to StoreData/1(DataFault) -> Terminator15/1
  Data collection chart/4(Sig_Vol_C123()) -> Terminator16/1
  Constant9/1 -> V_DUMP_CAN/1(count_in)
  V_DUMP_CAN/1(sig_trigger()) -> Subsystem/Trigger
  Constant10/1 -> Chart2/1(count_in)
  Chart2/1(sig_trigger()) -> Subsystem1/Trigger
  Chart3/1(sig_DMAInit_trigger()) -> DMA_Init/Trigger
  Constant11/1 -> Chart3/1(count_in)
  Constant12/1 -> Chart3/2(DMA_RST)
  Chart4/1(sig_KFInit_trigger()) -> SOCKF_Init1/Trigger
  Constant13/1 -> Chart4/1(count_in)
  Constant14/1 -> Chart4/2(KF_RST)
  Chart4/2(sig_KF_trigger()) -> SOCKF_Run/Trigger
  Constant15/1 -> Chart5/1(count_in)
  Chart5/1(sig_trigger()) -> Subsystem2/Trigger
  Chart/3(sig_trigger()) -> Subsystem3/Trigger
  Constant16/1 -> T_DUMP_CAN/1(count_in)
  T_DUMP_CAN/1(sig_trigger()) -> Subsystem4/Trigger
  RawData to StoreData (SPICh1)/1(DataFault) -> Terminator8/1
  S-Function Builder5/1 -> Terminator17/1, RawData to StoreData (SPICh1)/2(SPIData)
  S-Function Builder5/2 -> Terminator18/1, RawData to StoreData (SPICh1)/3(PecChk)

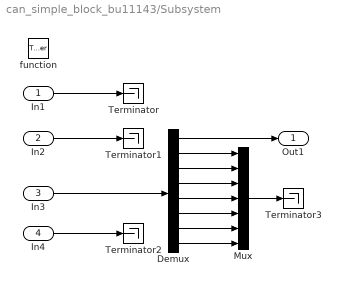
== system can_simple_block_bu11143/Subsystem ==
  In1 : Inport
  In2 : Inport  Port=2
  In3 : Inport  Port=3
  In4 : Inport  Port=4
  function : TriggerPort  TriggerType=function-call  VariantControl=Variant
  Demux : Demux  Outputs=8
  Mux : Mux  Inputs=7
  Terminator{,1..3} (4 alike) : Terminator
  Out1 : Outport
  wires:
  In1/1 -> Terminator/1
  In2/1 -> Terminator1/1
  In4/1 -> Terminator2/1
  In3/1 -> Demux/1
  Demux/8 -> Mux/7
  Demux/7 -> Mux/6
  Demux/6 -> Mux/5
  Demux/5 -> Mux/4
  Demux/4 -> Mux/3
  Demux/3 -> Mux/2
  Demux/2 -> Mux/1
  Mux/1 -> Terminator3/1
  Demux/1 -> Out1/1

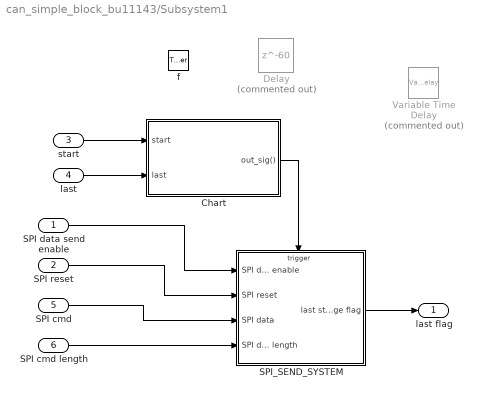
== system can_simple_block_bu11143/Subsystem1 ==
  SPI data send enable : Inport
  SPI reset : Inport  Port=2
  start : Inport  Port=3
  last : Inport  Port=4
  SPI cmd : Inport  Port=5
  SPI cmd length : Inport  Port=6
  f : TriggerPort  TriggerType=function-call  VariantControl=Variant
  Chart : Stateflow chart  TreatAsAtomicUnit=on
  Delay : Delay  Commented=on  DelayLength=60  InitialCondition=0
  SPI_SEND_SYSTEM : Subsystem
  Variable Time Delay : VariableTransportDelay  Commented=on  MaximumDelay=10
  last flag : Outport
  wires:
  SPI data send enable/1 -> SPI_SEND_SYSTEM/1(SPI data send enable)
  SPI reset/1 -> SPI_SEND_SYSTEM/2(SPI reset)
  SPI_SEND_SYSTEM/1(last stage flag) -> last flag/1
  start/1 -> Chart/1(start)
  last/1 -> Chart/2(last)
  SPI cmd/1 -> SPI_SEND_SYSTEM/3(SPI data)
  SPI cmd length/1 -> SPI_SEND_SYSTEM/4(SPI data length)
  Chart/1(out_sig()) -> SPI_SEND_SYSTEM/Trigger

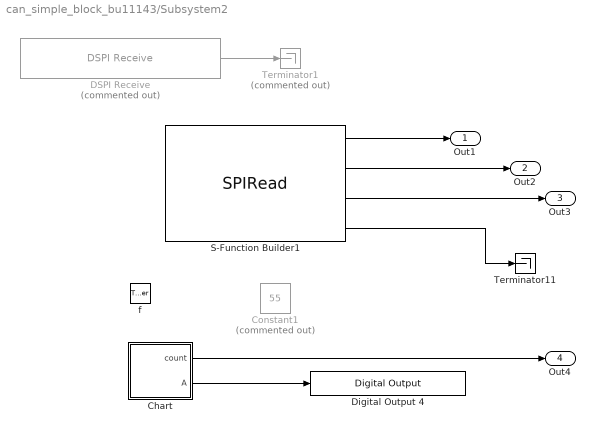
== system can_simple_block_bu11143/Subsystem2 ==
  f : TriggerPort  TriggerType=function-call  VariantControl=Variant
  Chart : Stateflow chart  TreatAsAtomicUnit=on
  Constant1 : Constant  Commented=on  Value=55  OutDataTypeStr=uint16
  DSPI Receive : rappid_564xl_ec_toolbox/MPC564xL/Communication Blocks/DSPI Receive  Commented=on  dspi_Num=1
  Digital Output 4 : rappid_564xl_ec_toolbox/MPC564xL/General Purpose Blocks/Digital Output   gpio_outputs="12  : PA12 : [ 122 ] : [ A10 ]"  pinNum=[ 122 ]  pcrNum=12
  S-Function Builder1 : S-Function  InitFcn=try, set_param(gcb,'FunctionName','SPIRead'), end  FunctionName=SPIRead  SFunctionModules=SPIRead_wrapper BMU_Driver  SFunctionDeploymentMode=off  EnableBusSupport=off  mask(S-Function Builder){}
      mask help: Simulink:masks:SFunctionBuilder_MD
      mask init: same as can_simple_block_bu11143/Function-Call Subsystem/S-Function Builder
      settings: CopyFcn=set_param(gcbh,'LinkStatus','none')  PreSaveFcn=try, set_param(gcb,'FunctionName','SPIRead'), end  OpenFcn=sfunctionwizard(gcbh)
      mask Display: plot(val(:,1),val(:,2)),disp(sys), port_label('output',1,'Vc1'), port_label('output',2,'Vc2'), port_label('output',3,'Vc3'), port_label('output',4,'PEC')
  Terminator1 : Terminator  Commented=on
  Terminator11 : Terminator
  Out1 : Outport
  Out2 : Outport  Port=2
  Out3 : Outport  Port=3
  Out4 : Outport  Port=4
  wires:
  Chart/2(" A") -> Digital Output 4/1
  Chart/1(count) -> Out4/1
  DSPI Receive/1 -> Terminator1/1
  S-Function Builder1/1 -> Out1/1
  S-Function Builder1/2 -> Out2/1
  S-Function Builder1/3 -> Out3/1
  S-Function Builder1/4 -> Terminator11/1

== system can_simple_block_bu11143/Subsystem3 ==
  start : Inport
  last : Inport  Port=2
  f : TriggerPort  TriggerType=function-call  VariantControl=Variant
  Chart : Stateflow chart  TreatAsAtomicUnit=on
  Out1 : Outport
  wires:
  start/1 -> Chart/1(start)
  last/1 -> Chart/2(last)
  Chart/1(out_sig()) -> Out1/1

== system can_simple_block_bu11143/Subsystem4 ==
  In1 : Inport
  f : TriggerPort  TriggerType=function-call  VariantControl=Variant
  Chart : Stateflow chart  TreatAsAtomicUnit=on
  DSPI Transmit : rappid_564xl_ec_toolbox/MPC564xL/Communication Blocks/DSPI Transmit  Priority=2  Commented=on  dspi_Num=0  dspi_CONT=off  dspi_PUSHR_PE=off  dspi_PUSHR_PP=off  dspi_PCS_0=36 : C[4] : [11] : [H3] : CS0  dspi_PCS_1=5 : A[5] : [14] : [H4] : CS0  dspi_PCS_2=3 : A[3] : [92] : [K17] : CS0  dspi_PCS_slave_0=36 : C[4] : [11] : [H3] : CS0  dspi_PCS_slave_1=5 : A[5] : [14] : [H4] : CS0  dspi_PCS_slave_2=3 : A[3] : [92] : [K17] : CS0  dspi_SIN_0=39 : C[7] : [15] : [K4] : SIN  dspi_SIN_1=8 : A[8] : [12] : [F4]  dspi_SIN_2=2 : A[2] : [84] : [N16] : SIN  dspi_SCK_0=37 : C[5] : [13] : [G3] : SCK  dspi_SCK_1=6 : A[6] : [2] : [G4] : SCK  dspi_SCK_2=0 : A[0] : [73] : [T14] : SCK  dspi_SOUT_0=38 : C[6] : [142] : [D4] : SOUT  dspi_SOUT_1=7 : A[7] : [10] : [F3] : SOUT  dspi_SOUT_2=1 : A[1] : [74] : [R14] : SOUT  dspi_Strobe=None  dspi_eoq=off  dspi_pcsx=Assert
  DSPI Transmit1 : rappid_564xl_ec_toolbox/MPC564xL/Communication Blocks/DSPI Transmit  Priority=2  Commented=on  dspi_Num=1  dspi_CONT=off  dspi_PUSHR_PE=off  dspi_PUSHR_PP=off  dspi_PCS_0=36 : C[4] : [11] : [H3] : CS0  dspi_PCS_1=105 : G[9] : [79] : [R17] : CS1  dspi_PCS_2=3 : A[3] : [92] : [K17] : CS0  dspi_PCS_slave_0=36 : C[4] : [11] : [H3] : CS0  dspi_PCS_slave_1=5 : A[5] : [14] : [H4] : CS0  dspi_PCS_slave_2=3 : A[3] : [92] : [K17] : CS0  dspi_SIN_0=39 : C[7] : [15] : [K4] : SIN  dspi_SIN_1=8 : A[8] : [12] : [F4]  dspi_SIN_2=2 : A[2] : [84] : [N16] : SIN  dspi_SCK_0=37 : C[5] : [13] : [G3] : SCK  dspi_SCK_1=6 : A[6] : [2] : [G4] : SCK  dspi_SCK_2=0 : A[0] : [73] : [T14] : SCK  dspi_SOUT_0=38 : C[6] : [142] : [D4] : SOUT  dspi_SOUT_1=7 : A[7] : [10] : [F3] : SOUT  dspi_SOUT_2=1 : A[1] : [74] : [R14] : SOUT  dspi_Strobe=None  dspi_eoq=off  dspi_pcsx=Assert
  Digital Output 1 : rappid_564xl_ec_toolbox/MPC564xL/General Purpose Blocks/Digital Output   gpio_outputs="79  : PE15 : [ 121 ] : [ B11 ]"  pinNum=[ 121 ]  pcrNum=79
  Terminator : Terminator
  Terminator1 : Terminator
  wires:
  In1/1 -> Terminator1/1
  Chart/1(count) -> Terminator/1
  Chart/2(" A") -> Digital Output 1/1

== system can_simple_block_bu11143/Function-Call Subsystem/DMA_Init ==
  function10ms : TriggerPort  TriggerType=function-call  VariantControl=Variant
  Data Type Conversion5 : DataTypeConversion  Priority=1  Commented=on
  S-Function Builder : S-Function  InitFcn=try, set_param(gcb,'FunctionName','DMA_init'), end  FunctionName=DMA_init  SFunctionModules=DMA_init_wrapper DMA  SFunctionDeploymentMode=off  EnableBusSupport=off  mask(S-Function Builder){}
      mask help: Simulink:masks:SFunctionBuilder_MD
      mask init: same as can_simple_block_bu11143/Function-Call Subsystem/S-Function Builder
      settings: CopyFcn=set_param(gcbh,'LinkStatus','none')  PreSaveFcn=try, set_param(gcb,'FunctionName','DMA_init'), end  OpenFcn=sfunctionwizard(gcbh)
      mask Display:
      | plot(val(:,1),val(:,2))
      | disp(sys)

== system can_simple_block_bu11143/Function-Call Subsystem/SOCKF_Init1 ==
  function10ms : TriggerPort  TriggerType=function-call  VariantControl=Variant
  Data Type Conversion5 : DataTypeConversion  Priority=1  Commented=on
  S-Function Builder1 : S-Function  InitFcn=try, set_param(gcb,'FunctionName','SOCEstimationInit'), end  FunctionName=SOCEstimationInit  SFunctionModules=SOCEstimationInit_wrapper Extended look2_binlx rtGetNaN rtGetInf rt_nonfinite const_params rt_roundd_snf  SFunctionDeploymentMode=off  EnableBusSupport=off  mask(S-Function Builder){}
      mask help: Simulink:masks:SFunctionBuilder_MD
      mask init: same as can_simple_block_bu11143/Function-Call Subsystem/S-Function Builder
      settings: CopyFcn=set_param(gcbh,'LinkStatus','none')  PreSaveFcn=try, set_param(gcb,'FunctionName','SOCEstimationInit'), end  OpenFcn=sfunctionwizard(gcbh)
      mask Display:
      | plot(val(:,1),val(:,2))
      | disp(sys)

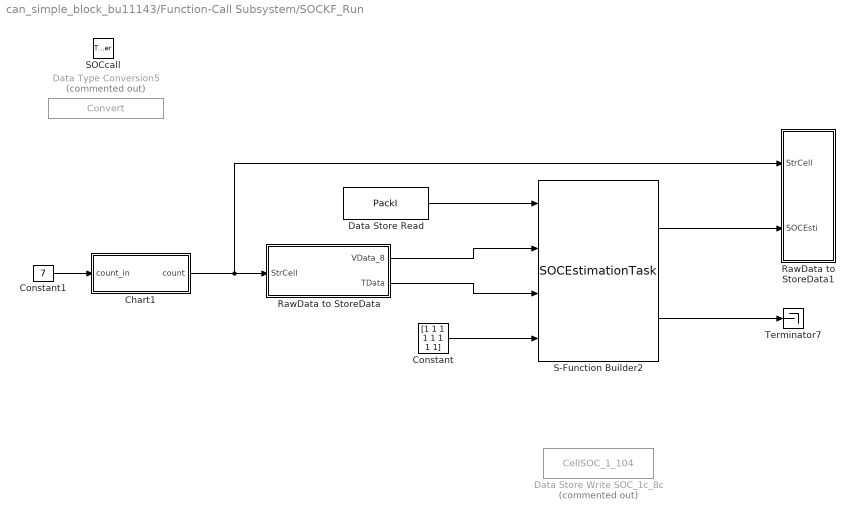
== system can_simple_block_bu11143/Function-Call Subsystem/SOCKF_Run ==
  SOCcall : TriggerPort  TriggerType=function-call  VariantControl=Variant
  Chart1 : Stateflow chart  TreatAsAtomicUnit=on
  Constant : Constant  Value=[1 1 1 1 1 1 1 1]  OutDataTypeStr=Inherit: Inherit via back propagation
  Constant1 : Constant  Value=7  OutDataTypeStr=uint8
  Data Store Read : DataStoreRead  DataStoreName=PackI
  Data Store Write SOC_1c_8c : DataStoreWrite  Commented=on  DataStoreName=CellSOC_1_104
  Data Type Conversion5 : DataTypeConversion  Priority=1  Commented=on
  RawData to StoreData : MATLAB Function  TreatAsAtomicUnit=on
  RawData to StoreData1 : MATLAB Function  TreatAsAtomicUnit=on
  S-Function Builder2 : S-Function  InitFcn=try, set_param(gcb,'FunctionName','SOCEstimationTask'), end  FunctionName=SOCEstimationTask  SFunctionModules=SOCEstimationTask_wrapper Extended look2_binlx rtGetNaN rtGetInf rt_nonfinite const_params rt_roundd_snf  SFunctionDeploymentMode=off  EnableBusSupport=off  mask(S-Function Builder){}
      mask help: Simulink:masks:SFunctionBuilder_MD
      mask init: same as can_simple_block_bu11143/Function-Call Subsystem/S-Function Builder
      settings: CopyFcn=set_param(gcbh,'LinkStatus','none')  PreSaveFcn=try, set_param(gcb,'FunctionName','SOCEstimationTask'), end  OpenFcn=sfunctionwizard(gcbh)
      mask Display:
      | plot(val(:,1),val(:,2))
      | disp(sys)
      | port_label('input',1,'I')
      | port_label('input',2,'V8')
      | port_label('input',3,'T')
      | port_label('input',4,'Enable8')
      | port_label('output',1,'SOC')
      | port_label('output',2,'Vt')
  Terminator7 : Terminator
  wires:
  Constant1/1 -> Chart1/1(count_in)
  Chart1/1(count) -> RawData to StoreData1/1(StrCell), RawData to StoreData/1(StrCell)
  RawData to StoreData/1(VData_8) -> S-Function Builder2/2
  Data Store Read/1 -> S-Function Builder2/1
  RawData to StoreData/2(TData) -> S-Function Builder2/3
  Constant/1 -> S-Function Builder2/4
  S-Function Builder2/1 -> RawData to StoreData1/2(SOCEsti)
  S-Function Builder2/2 -> Terminator7/1

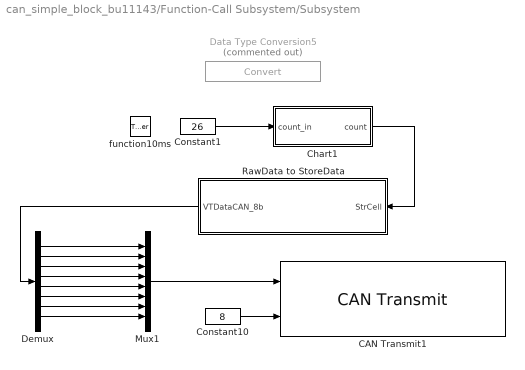
== system can_simple_block_bu11143/Function-Call Subsystem/Subsystem ==
  function10ms : TriggerPort  TriggerType=function-call  VariantControl=Variant
  CAN Transmit1 : rappid_564xl_ec_toolbox/MPC564xL/Communication Blocks/CAN Transmit  can_unit=A  can_unit_v2=0  can_buffer=14  can_id=522
  Chart1 : Stateflow chart  TreatAsAtomicUnit=on
  Constant1 : Constant  Value=26  OutDataTypeStr=uint8
  Constant10 : Constant  Value=8  OutDataTypeStr=uint8
  Data Type Conversion5 : DataTypeConversion  Priority=1  Commented=on
  Demux : Demux  Outputs=8
  Mux1 : Mux  Inputs=8
  RawData to StoreData : MATLAB Function  TreatAsAtomicUnit=on
  wires:
  Constant10/1 -> CAN Transmit1/2
  RawData to StoreData/1(VTDataCAN_8b) -> Demux/1
  Constant1/1 -> Chart1/1(count_in)
  Chart1/1(count) -> RawData to StoreData/1(StrCell)
  Demux/1 -> Mux1/1
  Demux/2 -> Mux1/2
  Demux/3 -> Mux1/3
  Demux/4 -> Mux1/4
  Demux/5 -> Mux1/5
  Demux/6 -> Mux1/6
  Demux/8 -> Mux1/8
  Demux/7 -> Mux1/7
  Mux1/1 -> CAN Transmit1/1
